simulink model "M2_1GDL"  (Simulink 9.1)
settings: Solver=ode45  StartTime=0.0  StopTime=10.0  FixedStep=.001  MaxStep=.0001  RelTol=1e-3  EnableMultiTasking=on
undefined symbols (not defined in the file or in its folder): bp, cp, denfc, hp, Im_pwm, Km2, numfc, p_pwm, Vp_pwm, Vtrasdp_ctp, z_ctp, zcomp, zp
settings Model: Creator=FEDERICA  LastModifiedBy=FEDERICA
settings DataIOCC: LimitDataPoints=on  SignalLoggingSaveFormat=ModelDataLogs
settings OptimizationCC: BlockReduction=off  BooleanDataType=off  LifeSpan=auto
settings DebuggingCC: SaveWithParameterizedLinksMsg=none  SignalResolutionControl=TryResolveAllWithWarning  MultiTaskDSMMsg=warning  MultiTaskCondExecSysMsg=none  SFUnexpectedBacktrackingDiag=error  SFNoUnconditionalDefaultTransitionDiag=error  SFExecutionAtInitializationDiag=warning
settings HardwareCC: ProdBitPerPointer=64  ProdBitPerSizeT=64  ProdBitPerPtrDiffT=64  ProdLargestAtomicFloat=Float  ProdIntDivRoundTo=Zero  ProdEndianess=LittleEndian  ProdWordSize=64  ProdHWDeviceType=Intel->x86-64 (Windows64)  TargetUnknown=on
settings CodeAppCC: StateflowObjectComments=off
settings ConfigComp: CovMetricSettings=dwe

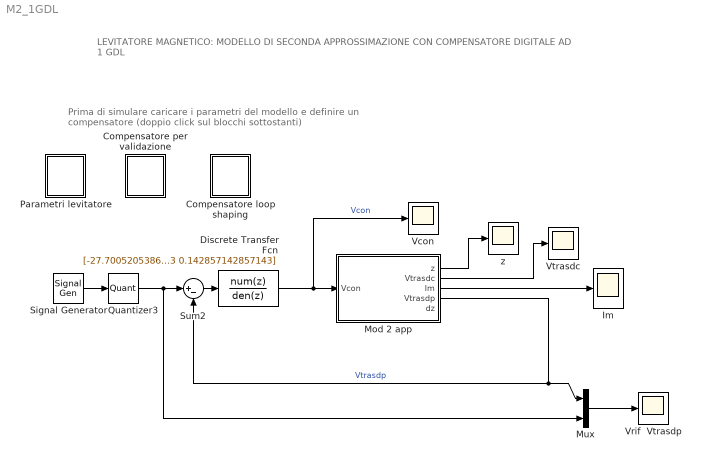
== system M2_1GDL ==
  note: LEVITATORE MAGNETICO: MODELLO DI SECONDA APPROSSIMAZIONE
      | CON COMPENSATORE DIGITALE AD 1 GDL
  note: Prima di simulare caricare i parametri del modello
      | e definire un compensatore (doppio click sul blocchi sottostanti)
  Compensatore loop shaping : Subsystem
      settings: OpenFcn=|
      | levitatore_m1
      | mod_lineare
      | loops
  Compensatore per validazione : Subsystem
      settings: OpenFcn=comp_base
  Discrete Transfer Fcn : DiscreteTransferFcn  Numerator=[-27.700520538613791 53.533590254399691 -25.864543606058280]  Denominator=[1 -1.142857142857143 0.142857142857143]  SampleTime=.001
  Im : Scope
  Mod 2 app : Subsystem  mask{Parameter1=0}
      mask prompts: Parameter1 "Mask Parameter 1:"
      mask Display:
      | port_label('input',1,'Vcon')
      | port_label('output',1,'z')
      | port_label('output',2,'Vtrasdc')
      | port_label('output',3,'Im')
      | port_label('output',4,'Vtrasdp')
      | port_label('output',5,'dz')
      | disp('M2')
  Mux : Mux  Inputs=2
  Parametri levitatore : Subsystem
      settings: OpenFcn=levitatore_m2
  Quantizer3 : Quantizer  QuantizationInterval=5e-3
  Signal Generator : SignalGenerator  WaveForm=sawtooth  Amplitude=-1  Frequency=.5
  Sum2 : Sum  Inputs=|+-  SaturateOnIntegerOverflow=on  InputSameDT=on  OutDataTypeStr=Inherit: Same as first input
  Vcon : Scope
  Vrif  Vtrasdp : Scope
  Vtrasdc : Scope
  z : Scope
  wires:
  Discrete Transfer Fcn/1 -> Vcon/1, Mod 2 app/1(Vcon)  "Vcon"
  Sum2/1 -> Discrete Transfer Fcn/1
  Signal Generator/1 -> Quantizer3/1
  Mux/1 -> Vrif  Vtrasdp/1
  Mod 2 app/2(Vtrasdc) -> Vtrasdc/1
  Mod 2 app/3(Im) -> Im/1
  Mod 2 app/4(Vtrasdp) -> Mux/1, Sum2/2  "Vtrasdp"
  Quantizer3/1 -> Sum2/1, Mux/2
  Mod 2 app/1(z) -> z/1

== system M2_1GDL/Compensatore loop shaping ==

== system M2_1GDL/Compensatore per validazione ==

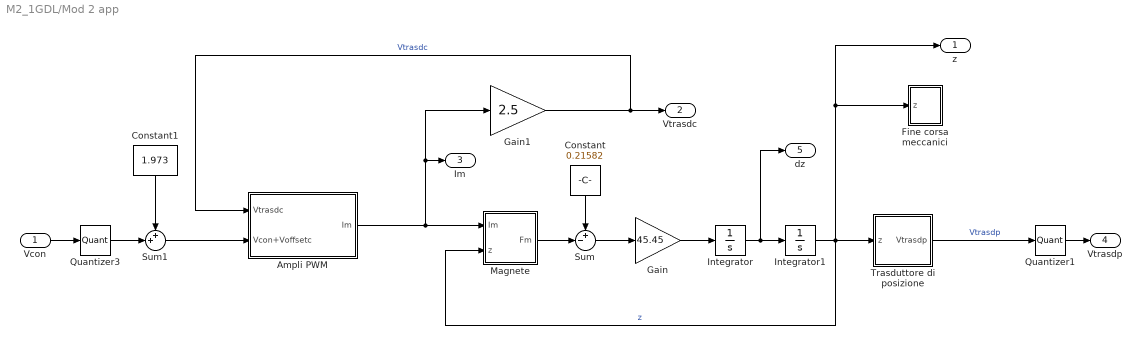
== system M2_1GDL/Mod 2 app ==
  Vcon : Inport
  Ampli PWM : Subsystem
  Constant : Constant  Value=0.21582
  Constant1 : Constant  Value=1.973
  Fine corsa meccanici : Subsystem
  Gain : Gain  Gain=45.45  SaturateOnIntegerOverflow=on  OutDataTypeStr=Inherit: Same as input  ParamDataTypeStr=Inherit: Same as input
  Gain1 : Gain  Gain=2.5  SaturateOnIntegerOverflow=on  OutDataTypeStr=Inherit: Same as input  ParamDataTypeStr=Inherit: Same as input
  Integrator : Integrator
  Integrator1 : Integrator  InitialCondition=0.02
  Magnete : Subsystem
  Quantizer1 : Quantizer  QuantizationInterval=5e-3
  Quantizer3 : Quantizer  QuantizationInterval=5e-3
  Sum : Sum  Inputs=+-|  SaturateOnIntegerOverflow=on  InputSameDT=on  OutDataTypeStr=Inherit: Same as first input
  Sum1 : Sum  Inputs=++|  SaturateOnIntegerOverflow=on  InputSameDT=on  OutDataTypeStr=Inherit: Same as first input
  Trasduttore di posizione : Subsystem
  z : Outport
  Vtrasdc : Outport  Port=2
  Im : Outport  Port=3
  Vtrasdp : Outport  Port=4
  dz : Outport  Port=5
  wires:
  Vcon/1 -> Quantizer3/1
  Quantizer3/1 -> Sum1/2
  Quantizer1/1 -> Vtrasdp/1
  Magnete/1(Fm) -> Sum/2
  Trasduttore di posizione/1(Vtrasdp) -> Quantizer1/1  "Vtrasdp"
  Ampli PWM/1(Im) -> Im/1, Gain1/1, Magnete/1(Im)
  Constant1/1 -> Sum1/1
  Sum1/1 -> Ampli PWM/2(Vcon+Voffsetc)
  Gain1/1 -> Vtrasdc/1, Ampli PWM/1(Vtrasdc)  "Vtrasdc"
  Integrator1/1 -> z/1, Fine corsa meccanici/1(z), Magnete/2(z), Trasduttore di posizione/1(z)  "z"
  Integrator/1 -> dz/1, Integrator1/1
  Gain/1 -> Integrator/1
  Sum/1 -> Gain/1
  Constant/1 -> Sum/1

== system M2_1GDL/Parametri levitatore ==

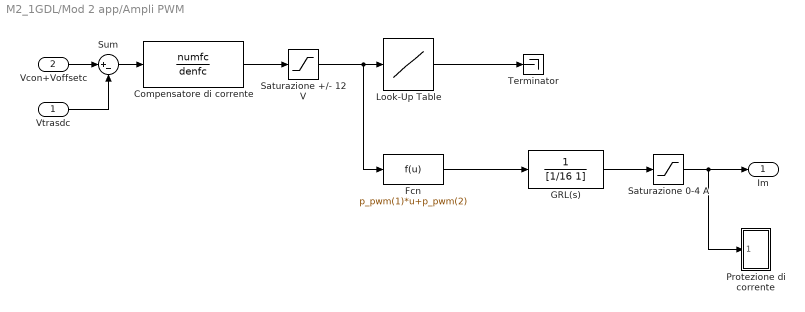
== system M2_1GDL/Mod 2 app/Ampli PWM ==
  Vtrasdc : Inport
  Vcon+Voffsetc : Inport  Port=2
  Compensatore di corrente : TransferFcn  Numerator=numfc  Denominator=denfc
  Fcn : Fcn  Expr=p_pwm(1)*u+p_pwm(2)
  GRL(s) : TransferFcn  Denominator=[1/16 1]
  Look-Up Table : Lookup  InputValues=Vp_pwm  Table=Im_pwm  SaturateOnIntegerOverflow=on
  Protezione di corrente : Subsystem
  Saturazione +/- 12 V : Saturate  UpperLimit=12  LowerLimit=-12
  Saturazione 0-4 A : Saturate  UpperLimit=4  LowerLimit=0
  Sum : Sum  Inputs=|+-  SaturateOnIntegerOverflow=on  InputSameDT=on  OutDataTypeStr=Inherit: Same as first input
  Terminator : Terminator
  Im : Outport
  wires:
  Look-Up Table/1 -> Terminator/1
  Compensatore di corrente/1 -> Saturazione +/- 12 V/1
  Vtrasdc/1 -> Sum/2
  Vcon+Voffsetc/1 -> Sum/1
  Sum/1 -> Compensatore di corrente/1
  Saturazione +/- 12 V/1 -> Fcn/1, Look-Up Table/1
  Fcn/1 -> GRL(s)/1
  GRL(s)/1 -> Saturazione 0-4 A/1
  Saturazione 0-4 A/1 -> Im/1, Protezione di corrente/1(Im)

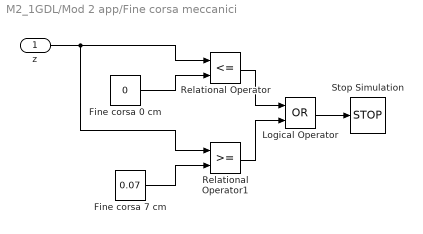
== system M2_1GDL/Mod 2 app/Fine corsa meccanici ==
  z : Inport
  Fine corsa 0 cm : Constant  Value=0
  Fine corsa 7 cm : Constant  Value=0.07
  Logical Operator : Logic  Operator=OR
  Relational Operator : RelationalOperator  Operator=<=  RndMeth=Nearest  InputSameDT=on
  Relational Operator1 : RelationalOperator  RndMeth=Nearest  InputSameDT=on
  Stop Simulation : Stop
  wires:
  Relational Operator1/1 -> Logical Operator/2
  Logical Operator/1 -> Stop Simulation/1
  z/1 -> Relational Operator1/1, Relational Operator/1
  Fine corsa 7 cm/1 -> Relational Operator1/2
  Fine corsa 0 cm/1 -> Relational Operator/2
  Relational Operator/1 -> Logical Operator/1

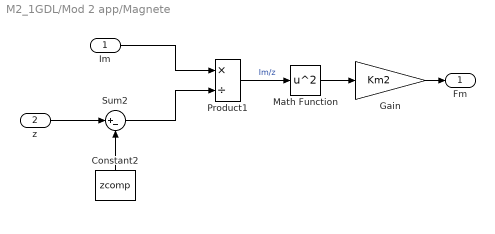
== system M2_1GDL/Mod 2 app/Magnete ==
  Im : Inport
  z : Inport  Port=2
  Constant2 : Constant  Value=zcomp
  Gain : Gain  Gain=Km2  SaturateOnIntegerOverflow=on  OutDataTypeStr=Inherit: Same as input  ParamDataTypeStr=Inherit: Same as input
  Math Function : Math  Operator=square  SaturateOnIntegerOverflow=on
  Product1 : Product  Inputs=*/  SaturateOnIntegerOverflow=on  RndMeth=Zero  InputSameDT=on  OutDataTypeStr=Inherit: Same as first input
  Sum2 : Sum  Inputs=|+-  SaturateOnIntegerOverflow=on  InputSameDT=on  OutDataTypeStr=Inherit: Same as first input
  Fm : Outport
  wires:
  Product1/1 -> Math Function/1  "Im/z"
  Sum2/1 -> Product1/2
  Constant2/1 -> Sum2/2
  z/1 -> Sum2/1
  Gain/1 -> Fm/1
  Math Function/1 -> Gain/1
  Im/1 -> Product1/1

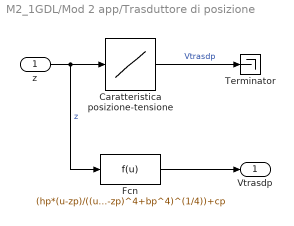
== system M2_1GDL/Mod 2 app/Trasduttore di posizione ==
  z : Inport
  Caratteristica posizione-tensione : Lookup  InputValues=flipud(z_ctp)  Table=flipud(Vtrasdp_ctp)  SaturateOnIntegerOverflow=on
  Fcn : Fcn  Expr=(hp*(u-zp)/((u-zp)^4+bp^4)^(1/4))+cp
  Terminator : Terminator
  Vtrasdp : Outport
  wires:
  Caratteristica posizione-tensione/1 -> Terminator/1  "Vtrasdp"
  Fcn/1 -> Vtrasdp/1
  z/1 -> Fcn/1, Caratteristica posizione-tensione/1  "z"

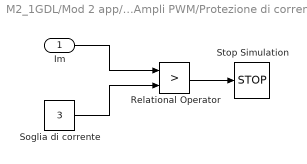
== system M2_1GDL/Mod 2 app/Ampli PWM/Protezione di corrente ==
  Im : Inport
  Relational Operator : RelationalOperator  Operator=>  RndMeth=Nearest  InputSameDT=on
  Soglia di corrente : Constant  Value=3
  Stop Simulation : Stop
  wires:
  Im/1 -> Relational Operator/1
  Relational Operator/1 -> Stop Simulation/1
  Soglia di corrente/1 -> Relational Operator/2
